simulink model "EPD629_WilliamsJ_AS12"  (R2021b)
settings: Solver=VariableStepAuto  StartTime=0.0  StopTime=45  MaxStep=0.0005  RelTol=1e-3
values from neighbouring files (symbols this model uses):
  AirMassFracO2 = 0.233    [EPD629_HW12_init.m]
  BPVAreaBreakpoints_pct = BPVAreaData_pct    [EPD629_HW12_init.m]
  BPVAreaData_pct = EGRValveAreaData_pct    [EPD629_HW12_init.m]
  BPVPositionBreakpoints_pct = EGRValvePositionBreakpoints_pct    [EPD629_HW12_init.m]
  BPVPositionData_pct = BPVPositionBreakpoints_pct    [EPD629_HW12_init.m]
  BPVWideOpenArea_mm2 = pi * BPVDiameter_mm^2 / 4    (= 7853.98163397)    [EPD629_HW12_init.m]
  CACDischargeCoefficient_frac = 0.7    [EPD629_HW12_init.m]
  CACEffectivenessData_frac = [1 0.95 0.92 0.885 0.87 0.85]    [EPD629_HW12_init.m]
  CACEffectivenessMassFlowBP_gps = [0 50 100 200 300 500]    [EPD629_HW12_init.m]
  CACFlowRestrictionArea_mm2 = 2000    [EPD629_HW12_init.m]
  CACVolume_L = 40    [EPD629_HW12_init.m]
  ClearanceVolumeTotal_L = 8/15    (= 0.533333333333)    [EPD629_HW12_init.m]
  Cp_cmp = 1.004    [EPD629_HW12_init.m]
  Cp_trb = 1.073    [EPD629_HW12_init.m]
  DesiredFuelBreakpoints_mg = 0:20:500    [EPD629_HW12_init.m]
  DischargeCoefficient_frac = 0.7    [EPD629_HW12_init.m]
  EGRCDischargeCoefficient_frac = 0.7    [EPD629_HW12_init.m]
  EGRCEffectivenessData_frac = [1 0.95 0.92 0.885 0.87 0.85]    [EPD629_HW12_init.m]
  EGRCEffectivenessMassFlowBP_gps = [0 50 100 200 300 500]    [EPD629_HW12_init.m]
  EGRCFlowRestrictionArea_mm2 = 500    [EPD629_HW12_init.m]
  EGRCoolerToValveVolume_L = 2    [EPD629_HW12_init.m]
  EGRValveAreaBreakpoints_pct = EGRValveAreaData_pct    [EPD629_HW12_init.m]
  EGRValveAreaData_pct = 100 * EGRValveArea_mm2 / EGRValveWideOpenArea_mm2    [EPD629_HW12_init.m]
  EGRValvePositionBreakpoints_pct = 0:100    [EPD629_HW12_init.m]
  EGRValvePositionData_pct = EGRValvePositionBreakpoints_pct    [EPD629_HW12_init.m]
  EGRValveWideOpenArea_mm2 = pi/4*50^2    (= 1963.49540849)    [EPD629_HW12_init.m]
  EngineDisplacement_L = 8    [EPD629_HW12_init.m]
  EngineSpeedBreakpoints_rpm = 600:200:3000    [EPD629_HW12_init.m]
  ExhaustManifoldGasConstant_kJpkgK = R_trb    (= 0.287)    [EPD629_HW12_init.m]
  ExhaustManifoldVolume_L = 8    [EPD629_HW12_init.m]
  FlowFunctionData_frac = PR.^(1/k_trb) .*      sqrt( 2 * k_trb / (k_trb - 1) .*      (1 - PR.^((k_trb - 1) / k_trb)) )    [EPD629_HW12_init.m]
  IntakeManifoldGasConstant_kJpkgK = Cp_im - Cv_im    (= 0.288)    [EPD629_HW12_init.m]
  IntakeManifoldVolume_L = 8    [EPD629_HW12_init.m]
  k_cmp = Cp_cmp/Cv_cmp    (= 1.40027894003)    [EPD629_HW12_init.m]
  k_trb = Cp_trb/Cv_trb    (= 1.36513994911)    [EPD629_HW12_init.m]
  ManifoldPressureBreakpoints_kPa = 80:20:500    [EPD629_HW12_init.m]
  NumberOfCylinders = 6    [EPD629_HW12_init.m]
  PressureRatioBreakpoints_frac = 0:0.01:1    [EPD629_HW12_init.m]
  R_cmp = Cp_cmp - Cv_cmp    (= 0.287)    [EPD629_HW12_init.m]
  R_trb = Cp_trb - Cv_trb    (= 0.287)    [EPD629_HW12_init.m]
  StoichiometricAFR_frac = 14.7    [EPD629_HW12_init.m]
  TurbineToBPVVolume_L = 10    [EPD629_HW12_init.m]
  TurbochargerInertia_kgm2 = 1e-4    (= 0.0001)    [EPD629_HW12_init.m]
  WastegateAreaData_pct = [0 100]    [EPD629_HW12_init.m]
  WastegateAreaGagePressBreakpoints_kPa = [250 300]    [EPD629_HW12_init.m]
  WastegateWideOpenArea_mm2 = pi/4*20^2    (= 314.159265359)    [EPD629_HW12_init.m]
undefined symbols (not defined in the file or in its folder): APPR_cmp, APPR_trb, ARPM_cmp, ARPM_trb, EFFI_cmp, EFFI_trb, ExhaustTemperatureData_degC, MASS_cmp, MASS_trb, MXRSP_cmp, MXRSP_trb, MXRVOL_cmp, MXRVOL_trb, PMAX_cmp, PMAX_trb, PMIN_cmp, PMIN_trb, ResidualCorrectionFactorData, VolumetricEfficiencyData_frac
libraries: simulink x2
(part 3 of 3)

== system EPD629_WilliamsJ_AS12/AirSystemPlantModel/TurbochargerFlow/TurboSpeed ==
  CompressorPower_kW : Inport
  TurbinePower_kW : Inport  Port=2
  Constant : Constant  Value=pi/30
  Constant1 : Constant  Value=TurbochargerInertia_kgm2
  Constant2 : Constant  Value=.03/pi
  Divide : Product  Inputs=*/
  Divide1 : Product  Inputs=*/
  Divide2 : Product  Inputs=**/
  Integrator : Integrator  InitialCondition=1  LimitOutput=on  UpperSaturationLimit=150  LowerSaturationLimit=1
  Product : Product
  Subtract : Sum  Inputs=+-
  TurboSpeed_krpm : Outport
  wires:
  Constant/1 -> Product/1
  CompressorPower_kW/1 -> Divide/1
  Divide/1 -> Subtract/2
  TurbinePower_kW/1 -> Divide1/1
  Divide1/1 -> Subtract/1
  Product/1 -> Divide1/2, Divide/2
  Subtract/1 -> Divide2/2  "N*m"
  Constant1/1 -> Divide2/3
  Constant2/1 -> Divide2/1
  Divide2/1 -> Integrator/1
  Integrator/1 -> Product/2, TurboSpeed_krpm/1

== system EPD629_WilliamsJ_AS12/VirtualSensor/EngineFlow/CylinderEVO ==
  CylinderIVCMassAir_mg : Inport
  CylinderIVCMass_mg : Inport  Port=2
  EngineSpeed_rpm : Inport  Port=3
  CylinderResidualMass_mg : Inport  Port=4
  DesiredFuel_mg : Inport  Port=5
  Add1 : Sum  Inputs=+-
  Add6 : Sum  Inputs=+-
  Add7 : Sum  Inputs=2
  Constant1 : Constant  Value=AirMassFracO2
  Constant13 : Constant  Value=StoichiometricAFR_frac
  Constant2 : Constant  Value=StoichiometricAFR_frac
  Constant5 : Constant  Value=NumberOfCylinders
  Constant6 : Constant  Value=120000
  Max1 : MinMax  Inputs=2
  Max6 : MinMax  Function=max  Inputs=2
  P_a4 : Constant
  Product1 : Product  RndMeth=Zero
  Product11 : Product  Inputs=*/  RndMeth=Zero
  Product13 : Product  Inputs=*/  RndMeth=Zero
  Product14 : Product  RndMeth=Zero
  Product3 : Product  Inputs=***/  RndMeth=Zero
  CylindersOutMassFlow_gps : Outport
  CylindersOutMassFracO2 : Outport  Port=2
  CombustionMassFuel_mg : Outport  Port=3
  wires:
  Product1/1 -> Add6/2  "CombustionMassAir_mg"
  Max1/1 -> Product1/1, CombustionMassFuel_mg/1  "CombustionMassFuel_mg"
  Constant2/1 -> Product1/2
  CylinderIVCMass_mg/1 -> Add7/2
  EngineSpeed_rpm/1 -> Product3/2
  P_a4/1 -> Max6/2
  Product11/1 -> Max1/2  "StoichiometricFuelMass_mg"
  Constant13/1 -> Product11/2
  Constant1/1 -> Product14/2
  Add7/1 -> Max6/1, Add1/1  "CylinderEVOMass_mg"
  Constant5/1 -> Product3/3
  Product14/1 -> Product13/1  "CylinderEVOMassO2_mg"
  Add6/1 -> Product14/1  "CylinderEVOMassAir_mg"
  Product13/1 -> CylindersOutMassFracO2/1
  CylinderIVCMassAir_mg/1 -> Add6/1, Product11/1
  Constant6/1 -> Product3/4
  Max6/1 -> Product13/2
  Product3/1 -> CylindersOutMassFlow_gps/1
  DesiredFuel_mg/1 -> Max1/1, Add7/1
  CylinderResidualMass_mg/1 -> Add1/2
  Add1/1 -> Product3/1  "CylinderOutMass_mg"

== system EPD629_WilliamsJ_AS12/VirtualSensor/EngineFlow/CylinderIVC ==
  CylinderInMass_mg : Inport
  IntakeManifoldMassFracO2 : Inport  Port=2
  CylinderResidualMass_mg : Inport  Port=3
  CylindersOutMassFracO2 : Inport  Port=4
  Add4 : Sum  Inputs=2
  Add5 : Sum
  Constant1 : Constant  Value=AirMassFracO2
  Max4 : MinMax  Function=max  Inputs=2
  P_a1 : Constant
  Product10 : Product  Inputs=*/  RndMeth=Zero
  Product7 : Product  RndMeth=Zero
  Product8 : Product  Inputs=*/  RndMeth=Zero
  Product9 : Product  RndMeth=Zero
  CylinderResidualMassO2_mg : Outport
  CylinderIVCMassFracO2 : Outport  Port=2
  CylinderIVCMassAir_mg : Outport  Port=3
  CylinderIVCMass_mg : Outport  Port=4
  wires:
  P_a1/1 -> Max4/1
  Product10/1 -> CylinderIVCMassAir_mg/1
  Constant1/1 -> Product10/2
  CylindersOutMassFracO2/1 -> Product9/2
  Add4/1 -> CylinderIVCMass_mg/1, Max4/2  "CylinderIVCMass_mg"
  CylinderResidualMass_mg/1 -> Product9/1, Add4/1
  Product8/1 -> CylinderIVCMassFracO2/1
  Product7/1 -> Add5/2  "CylinderInMassO2_mg"
  Product9/1 -> Add5/1, CylinderResidualMassO2_mg/1  "CylinderResidualMassO2_mg"
  Add5/1 -> Product10/1, Product8/1  "CylinderIVCMassO2_mg"
  CylinderInMass_mg/1 -> Product7/1, Add4/2
  Max4/1 -> Product8/2
  IntakeManifoldMassFracO2/1 -> Product7/2

== system EPD629_WilliamsJ_AS12/VirtualSensor/EngineFlow/ExhaustTempAndResidualMass ==
  note: K
  note: kg/m^3
      | g/L
  note: kJ/(kg*K)
  note: kPa
  note: mg/g
  EngineSpeed_rpm : Inport
  ExhaustManifoldPress_kPa : Inport  Port=2
  CombustionMassFuel_mg : Inport  Port=3
  Add3 : Sum
  Constant1 : Constant  Value=NumberOfCylinders
  Constant10 : Constant  Value=ExhaustManifoldGasConstant_kJpkgK
  Constant11 : Constant
  Constant12 : Constant  Value=1000
  Constant8 : Constant  Value=ClearanceVolumeTotal_L
  Constant9 : Constant  Value=273.15
  ExhaustTemperatureData_degC : Lookup_n-D  BreakpointsForDimension1=DesiredFuelBreakpoints_mg  BreakpointsForDimension2=EngineSpeedBreakpoints_rpm  Table=ExhaustTemperatureData_degC  ExtrapMethod=Clip  UseLastTableValue=on  InternalRulePriority=Speed  RndMeth=Simplest  InputSameDT=on
      settings: InputPortMap=u0,u1
  Max3 : MinMax  Function=max  Inputs=2
  Product5 : Product  Inputs=*//  RndMeth=Zero
  Product6 : Product  Inputs=****/  RndMeth=Zero
  ResidualCorrectionFactorData : Lookup_n-D  BreakpointsForDimension1=DesiredFuelBreakpoints_mg  BreakpointsForDimension2=EngineSpeedBreakpoints_rpm  Table=ResidualCorrectionFactorData  ExtrapMethod=Clip  UseLastTableValue=on  InternalRulePriority=Speed  RndMeth=Simplest  InputSameDT=on
      settings: InputPortMap=u0,u1
  CylinderResidualMass_mg : Outport
  CylindersOutTemp_degC : Outport  Port=2
  wires:
  ResidualCorrectionFactorData/1 -> Product6/3
  Constant12/1 -> Product6/1
  Constant1/1 -> Product6/5
  Constant9/1 -> Add3/1
  EngineSpeed_rpm/1 -> ExhaustTemperatureData_degC/2, ResidualCorrectionFactorData/2
  CombustionMassFuel_mg/1 -> ExhaustTemperatureData_degC/1, ResidualCorrectionFactorData/1
  Product5/1 -> Product6/2  "ExhaustManifoldDensity_gpL"
  Max3/1 -> Product5/3
  Product6/1 -> CylinderResidualMass_mg/1
  ExhaustManifoldPress_kPa/1 -> Product5/1
  Constant11/1 -> Max3/2
  Add3/1 -> Max3/1
  Constant10/1 -> Product5/2
  ExhaustTemperatureData_degC/1 -> CylindersOutTemp_degC/1, Add3/2
  Constant8/1 -> Product6/4

== system EPD629_WilliamsJ_AS12/VirtualSensor/EngineFlow/SpeedDensityMassFlow ==
  note: g
  note: mg/g
  note: K
  note: kg/m^3
      | g/L
  note: kJ/(kg*K)
  note: L
  note: kPa
  IntakeManifoldPress_kPa : Inport
  IntakeManifoldTemp_degC : Inport  Port=2
  EngineSpeed_rpm : Inport  Port=3
  Add1 : Sum
  Constant : Constant  Value=273.15
  Constant2 : Constant  Value=IntakeManifoldGasConstant_kJpkgK
  Constant3 : Constant  Value=EngineDisplacement_L
  Constant4 : Constant
  Constant7 : Constant  Value=NumberOfCylinders
  Max2 : MinMax  Function=max  Inputs=2
  P_a3 : Constant  Value=1000
  Product1 : Product  Inputs=*//  RndMeth=Zero
  Product2 : Product  Inputs=3  RndMeth=Zero
  Product3 : Product
  Product4 : Product  Inputs=**/
  VolumetricEfficiencyData_frac : Lookup_n-D  BreakpointsForDimension1=ManifoldPressureBreakpoints_kPa  BreakpointsForDimension2=EngineSpeedBreakpoints_rpm  Table=VolumetricEfficiencyData_frac  ExtrapMethod=Clip  UseLastTableValue=on  InternalRulePriority=Speed  RndMeth=Simplest  InputSameDT=on
      settings: InputPortMap=u0,u1
  rpm to cycles/sec : Gain  Gain=1/120
  SpeedDensityMassFlow_gps : Outport
  CylinderInMass_mg : Outport  Port=2
  wires:
  Product3/1 -> SpeedDensityMassFlow_gps/1
  Product2/1 -> Product4/2, Product3/2
  Constant7/1 -> Product4/3
  Product4/1 -> CylinderInMass_mg/1
  P_a3/1 -> Product4/1
  Constant2/1 -> Product1/2
  VolumetricEfficiencyData_frac/1 -> Product2/3  "VolumetricEfficiency_frac"
  Constant4/1 -> Max2/2
  Add1/1 -> Max2/1
  IntakeManifoldTemp_degC/1 -> Add1/1
  IntakeManifoldPress_kPa/1 -> VolumetricEfficiencyData_frac/1, Product1/1
  Constant3/1 -> Product2/2
  rpm to cycles/sec/1 -> Product3/1
  Max2/1 -> Product1/3
  Product1/1 -> Product2/1  "IntakeManifoldDensity_gpL"
  Constant/1 -> Add1/2
  EngineSpeed_rpm/1 -> VolumetricEfficiencyData_frac/2, rpm to cycles/sec/1
